simulink subsystem "MountModel"  (R2022b)
settings: Solver=VariableStepAuto  StartTime=0.0  StopTime=10.0  RelTol=1e-3
settings Model: Creator=kevin  LastModifiedBy=kevin

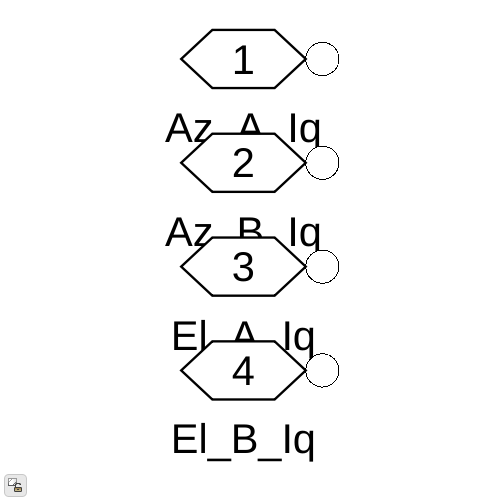
[thumbnail: Simulink's stored preview of the top-level diagram]
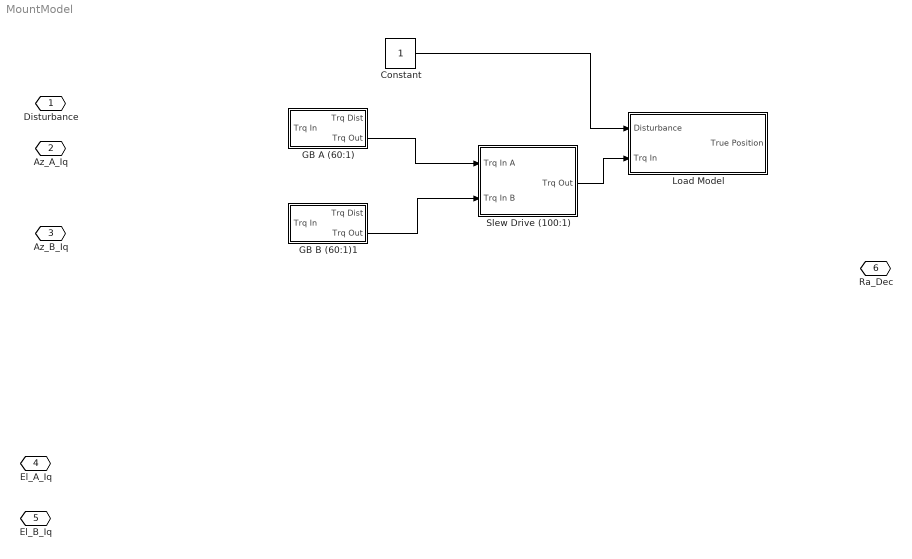
== system MountModel ==
  Constant : Constant
  GB A (60:1) : Subsystem
  GB B (60:1)1 : Subsystem
  Load Model : Subsystem
  Slew Drive (100:1) : Subsystem
  Disturbance : PMIOPort  Side=Left
  Az_A_Iq : PMIOPort  Port=2  Side=Left
  Az_B_Iq : PMIOPort  Port=3  Side=Left
  El_A_Iq : PMIOPort  Port=4  Side=Left
  El_B_Iq : PMIOPort  Port=5  Side=Left
  Ra_Dec : PMIOPort  Port=6  Side=Right
  wires:
  GB A (60:1)/2(Trq Out) -> Slew Drive (100:1)/1(Trq In A)
  Constant/1 -> Load Model/1(Disturbance)
  GB B (60:1)1/2(Trq Out) -> Slew Drive (100:1)/2(Trq In B)
  Slew Drive (100:1)/1(Trq Out) -> Load Model/2(Trq In)

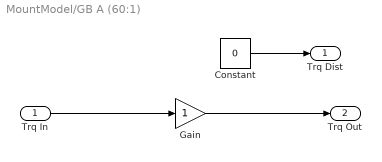
== system MountModel/GB A (60:1) ==
  Trq In : Inport
  Constant : Constant  Value=0
  Gain : Gain
  Trq Dist : Outport
  Trq Out : Outport  Port=2
  wires:
  Constant/1 -> Trq Dist/1
  Trq In/1 -> Gain/1
  Gain/1 -> Trq Out/1

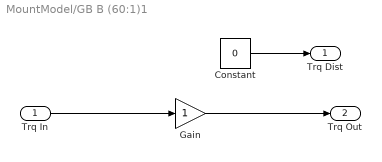
== system MountModel/GB B (60:1)1 ==
  Trq In : Inport
  Constant : Constant  Value=0
  Gain : Gain
  Trq Dist : Outport
  Trq Out : Outport  Port=2
  wires:
  Gain/1 -> Trq Out/1
  Trq In/1 -> Gain/1
  Constant/1 -> Trq Dist/1

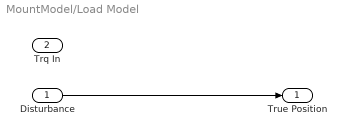
== system MountModel/Load Model ==
  Disturbance : Inport
  Trq In : Inport  Port=2
  True Position : Outport
  wires:
  Disturbance/1 -> True Position/1

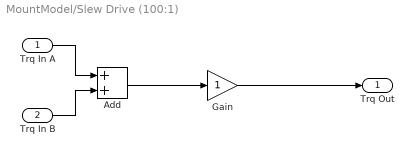
== system MountModel/Slew Drive (100:1) ==
  Trq In A : Inport
  Trq In B : Inport  Port=2
  Add : Sum
  Gain : Gain
  Trq Out : Outport
  wires:
  Add/1 -> Gain/1
  Trq In B/1 -> Add/2
  Gain/1 -> Trq Out/1
  Trq In A/1 -> Add/1
